simulink model "comp_model"  (R2013a)
settings: Solver=FixedStepDiscrete  StartTime=0.0  StopTime=3  RelTol=1e-3
undefined symbols (not defined in the file or in its folder): fdesignblkfcn, gcbh
libraries: xpcnilib x1
settings Model: BufferReuse=off  Creator=dholley  LastModifiedBy=dholley
settings OptimizationCC: BlockReduction=off  OptimizeBlockIOStorage=off  BufferReuse=off  ExpressionFolding=off  LocalBlockOutputs=off
settings HardwareCC: ProdIntDivRoundTo=Zero  ProdEndianess=LittleEndian  ProdHWDeviceType=Generic->32-bit x86 compatible
settings RTWCC: SystemTargetFile=xpctarget.tlc  TemplateMakefile=xpc_default_tmf  Description=xPC Target  ProcessScript=xpctarget_make_rtw_hook  RTWCompilerOptimization=On
settings xpcTargetCC: TargetFcnLib=ansi_tfl_table_tmw.mat  CodeReplacementLibrary=XPC_BLAS  ParMdlRefBuildCompliant=on  ConcurrentExecutionCompliant=on  CombineSignalStateStructs=off  MATLABClassNameForMDSCustomization=xpcAperiodicCustomization  GRTInterface=on  GenerateAllocFcn=off  xPCTaskExecutionProfile=off  xPCRL32EventNumber=5000  xPCLoadParamSetFile=off  xPCConcurrentTasks=off  xPCEnableSFAnimation=off

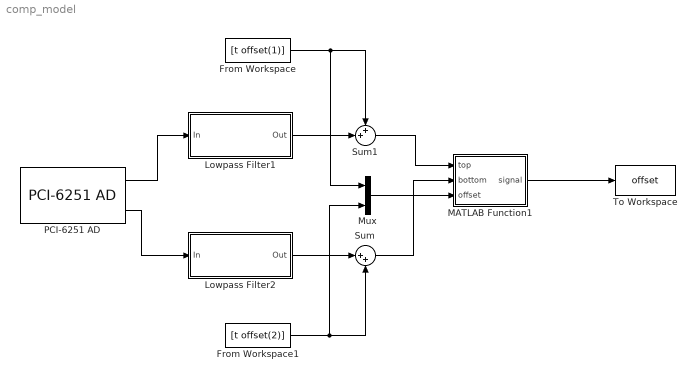
== system comp_model ==
  From Workspace : FromWorkspace  VariableName=[t offset(1)]  SampleTime=.001
  From Workspace1 : FromWorkspace  VariableName=[t offset(2)]  SampleTime=.001
  Lowpass Filter1 : Subsystem  DialogController=fdesignblkfcn  InitFcn=fdesignblkfcn(gcbh, {'InitFcn'});  mask(Lowpass Filter){}
      mask help: Design a lowpass filter
      settings: CopyFcn=fdesignblkfcn(gcbh, {'CopyFcn'});
      mask Help: helpview(mapfilelocation('dsp'), 'dsplowpassfilter');
      mask Display: disp('Lowpass')
  Lowpass Filter2 : Subsystem  DialogController=fdesignblkfcn  InitFcn=fdesignblkfcn(gcbh, {'InitFcn'});  mask(Lowpass Filter){}
      mask help: Design a lowpass filter
      settings: CopyFcn=fdesignblkfcn(gcbh, {'CopyFcn'});
      mask Help: helpview(mapfilelocation('dsp'), 'dsplowpassfilter');
      mask Display: disp('Lowpass')
  MATLAB Function1 : MATLAB Function  TreatAsAtomicUnit=on
  Mux : Mux  Inputs=2
  PCI-6251 AD : xpcnilib/A//D/M Series/PCI-6251 AD  channel=[7,8]  range=[5,5]  coupling=[2,2]  scantime=5e-6  sampletime=0.001  slot=-1
  Sum : Sum  Inputs=|++
  Sum1 : Sum  Inputs=++|
  To Workspace : ToWorkspace  VariableName=offset  SampleTime=.001  SaveFormat=Timeseries
  wires:
  PCI-6251 AD/1 -> Lowpass Filter1/1(In)
  PCI-6251 AD/2 -> Lowpass Filter2/1(In)
  MATLAB Function1/1(signal) -> To Workspace/1
  Lowpass Filter1/1(Out) -> Sum1/2
  Lowpass Filter2/1(Out) -> Sum/1
  Sum/1 -> MATLAB Function1/2(bottom)
  Sum1/1 -> MATLAB Function1/1(top)
  Mux/1 -> MATLAB Function1/3(offset)
  From Workspace1/1 -> Mux/2, Sum/2
  From Workspace/1 -> Mux/1, Sum1/1

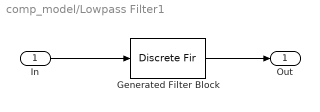
== system comp_model/Lowpass Filter1 ==
  In : Inport
  Generated Filter Block : DiscreteFir  Tag=BlockMethodSubSystem  Coefficients=[0.0035257793515495774 0.0038119531647798038 0.0041036148788394806 0.0044003780267683791 0.0047018389448218933 0.0050075775498282637 0.0053171581667394901 0.0056301304044040169 0.0059460300774376931 0.0062643801719234971 0.0065846918525311708 0.0069064655085147161 0.0072291918359202803 0.0075523529532183957 0.0078754235474644951 0.0081978720479896055 0.008519161824529782 0.008838752406618456 0.0091561007209909322 0.0094706623436844779 0.0097818927634617959 0.010089248653139572 0.010392189145368247 0.010690177109383412 0.010982680425234054 0.011269173251988259 0.011549137286422439 0.011822063008716528 0.012087450911703952 0.012344812710262444 0.01259367252747858 0.012833568054276996 0.013064051679271809 0.013284691585675896 0.013495072812189788 0.013694798274888394 0.013883489747229208 0.014060788795419015 0.014226357666499202 0.014379880126639598 0.014521062247269227 0.014649633136817507 0.014765345615991476 0.014867976834673335 0.014957328828686459 0.015033229014848307 0.015095530622902396 0.015144113063101152 0.015178882228393269 0.015199770730355538 0.015206738068197194 0.015199770730355538 0.015178882228393269 0.015144113063101152 0.015095530622902396 0.015033229014848307 0.014957328828686459 0.014867976834673335 0.014765345615991476 0.014649633136817507 0.014521062247269227 0.014379880126639598 0.014226357666499202 0.014060788795419015 0.013883489747229208 0.013694798274888394 0.013495072812189788 0.013284691585675896 0.013064051679271809 0.012833568054276996 0.01259367252747858 0.012344812710262444 0.012087450911703952 0.011822063008716528 0.011549137286422439 0.011269173251988259 0.010982680425234054 0.010690177109383412 0.010392189145368247 0.010089248653139572 0.0097818927634617959 0.0094706623436844779 0.0091561007209909322 0.008838752406618456 0.008519161824529782 0.0081978720479896055 0.0078754235474644951 0.0075523529532183957 0.0072291918359202803 0.0069064655085147161 0.0065846918525311708 0.0062643801719234971 0.0059460300774376931 0.0056301304044040169 0.0053171581667394901 0.0050075775498282637 0.0047018389448218933 0.0044003780267683791 0.0041036148788394806 0.0038119531647798038 0.0035257793515495774]  InputProcessing=Columns as channels (frame based)
  Out : Outport
  wires:
  In/1 -> Generated Filter Block/1
  Generated Filter Block/1 -> Out/1

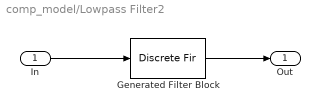
== system comp_model/Lowpass Filter2 ==
  In : Inport
  Generated Filter Block : DiscreteFir  Tag=BlockMethodSubSystem  Coefficients=[0.0035257793515495774 0.0038119531647798038 0.0041036148788394806 0.0044003780267683791 0.0047018389448218933 0.0050075775498282637 0.0053171581667394901 0.0056301304044040169 0.0059460300774376931 0.0062643801719234971 0.0065846918525311708 0.0069064655085147161 0.0072291918359202803 0.0075523529532183957 0.0078754235474644951 0.0081978720479896055 0.008519161824529782 0.008838752406618456 0.0091561007209909322 0.0094706623436844779 0.0097818927634617959 0.010089248653139572 0.010392189145368247 0.010690177109383412 0.010982680425234054 0.011269173251988259 0.011549137286422439 0.011822063008716528 0.012087450911703952 0.012344812710262444 0.01259367252747858 0.012833568054276996 0.013064051679271809 0.013284691585675896 0.013495072812189788 0.013694798274888394 0.013883489747229208 0.014060788795419015 0.014226357666499202 0.014379880126639598 0.014521062247269227 0.014649633136817507 0.014765345615991476 0.014867976834673335 0.014957328828686459 0.015033229014848307 0.015095530622902396 0.015144113063101152 0.015178882228393269 0.015199770730355538 0.015206738068197194 0.015199770730355538 0.015178882228393269 0.015144113063101152 0.015095530622902396 0.015033229014848307 0.014957328828686459 0.014867976834673335 0.014765345615991476 0.014649633136817507 0.014521062247269227 0.014379880126639598 0.014226357666499202 0.014060788795419015 0.013883489747229208 0.013694798274888394 0.013495072812189788 0.013284691585675896 0.013064051679271809 0.012833568054276996 0.01259367252747858 0.012344812710262444 0.012087450911703952 0.011822063008716528 0.011549137286422439 0.011269173251988259 0.010982680425234054 0.010690177109383412 0.010392189145368247 0.010089248653139572 0.0097818927634617959 0.0094706623436844779 0.0091561007209909322 0.008838752406618456 0.008519161824529782 0.0081978720479896055 0.0078754235474644951 0.0075523529532183957 0.0072291918359202803 0.0069064655085147161 0.0065846918525311708 0.0062643801719234971 0.0059460300774376931 0.0056301304044040169 0.0053171581667394901 0.0050075775498282637 0.0047018389448218933 0.0044003780267683791 0.0041036148788394806 0.0038119531647798038 0.0035257793515495774]  InputProcessing=Columns as channels (frame based)
  Out : Outport
  wires:
  In/1 -> Generated Filter Block/1
  Generated Filter Block/1 -> Out/1

== matlab function comp_model/MATLAB Function1 ==
  data: top input; signal output; bottom input; offset input
function signal = fcn(top,bottom,offset)
%#codegen

f1=zeros(3000,1);
f2=zeros(3000,1);

for i=1:3000
    f1(i)=top(i);
    f2(i)=bottom(i);
end

coder.extrinsic('questdlg','accept')

ftop=f1(200:end);
fbottom=f2(200:end);

caltop=mean(ftop);
calbottom=mean(fbottom);

accept=questdlg('Offset of \caltop and \calbottom detected. Proceed with bias?','Zero Calibration','Yes','No','Reset','Yes');
    
    switch accept
        case 'Yes'
            signal=[caltop calbottom];
        case 'No'
            signal=offset;
        case 'Reset'
            signal=[0 0];
    end
end
